simulink subsystem "Piero"  (R2022b)
settings: Solver=VariableStepAuto  StartTime=0.0  StopTime=10.0  RelTol=1e-3
settings Model: Creator=David  LastModifiedBy=dar.io

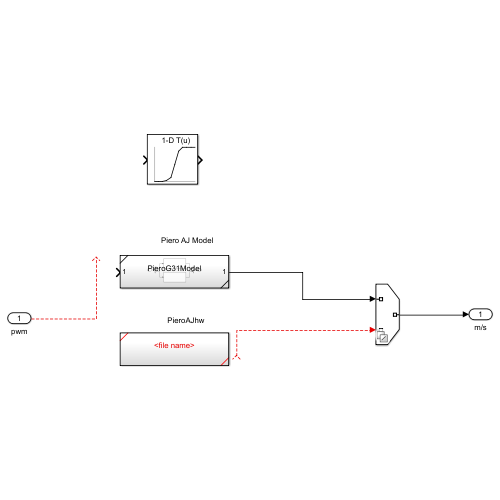
[thumbnail: Simulink's stored preview of the top-level diagram]
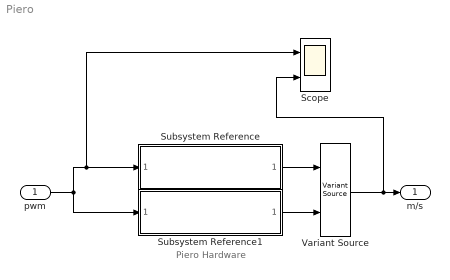
== system Piero ==
  note: Piero Hardware
  pwm : Inport
  Scope : Scope  NumInputPorts=2
  Subsystem Reference : Subsystem  ReferencedSubsystem=PieroG31Model
  Subsystem Reference1 : Subsystem  ReferencedSubsystem=PieroHW
  Variant Source : VariantSource  VariantControlMode=sim codegen switching
  m/s : Outport
  wires:
  Subsystem Reference1/1 -> Variant Source/2
  pwm/1 -> Subsystem Reference/1, Scope/1, Subsystem Reference1/1
  Variant Source/1 -> m/s/1, Scope/2
  Subsystem Reference/1 -> Variant Source/1
